simulink model "IIR_Filter_int32"  (R2018b)
settings: configuration reference "Test_PIL_IIR_Filter_config_ref" (kept outside this file)
settings Model: SimulationMode=processor-in-the-loop (pil)  Creator=reynaudp  LastModifiedBy=fenard1
settings ConfigSetRef: SourceLocation=Base Workspace

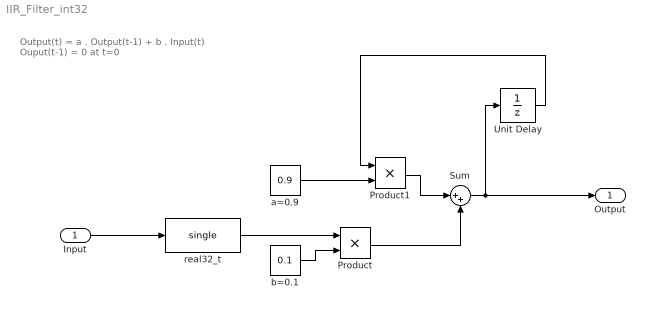
== system IIR_Filter_int32 ==
  note: Output(t) = a . Output(t-1) + b . Input(t)
      | Ouput(t-1) = 0 at t=0
  Input : Inport  OutDataTypeStr=int32  PortDimensions=1  SampleTime=0.001  Interpolate=off
  Product : Product  RndMeth=Zero  OutDataTypeStr=Inherit: Same as first input
  Product1 : Product  RndMeth=Zero  OutDataTypeStr=Inherit: Same as first input
  Sum : Sum  Inputs=|++  OutDataTypeStr=Inherit: Same as first input
  Unit Delay : UnitDelay  SampleTime=-1
  a=0.9 : Constant  Value=0.9  VectorParams1D=off  OutDataTypeStr=single
  b=0.1 : Constant  Value=0.1  OutDataTypeStr=single  LockScale=on
  real32_t : DataTypeConversion  OutDataTypeStr=single
  Output : Outport  OutDataTypeStr=single
  wires:
  Input/1 -> real32_t/1
  Unit Delay/1 -> Product1/1
  Product1/1 -> Sum/1
  Product/1 -> Sum/2
  b=0.1/1 -> Product/2
  a=0.9/1 -> Product1/2
  real32_t/1 -> Product/1
  Sum/1 -> Unit Delay/1, Output/1
